simulink model "observer_based_SF_controller"  (R2017b)
settings: Solver=VariableStepAuto  StartTime=0.0  StopTime=10.0  RelTol=1e-3
values from neighbouring files (symbols this model uses):
  mA = [0 1 0; 0 -b/j k/j; 0 k/l -r/l]    [ProjectFile1.m]
  mB = [0;0; 1/l]    [ProjectFile1.m]
  mC = [1 0 0]    [ProjectFile1.m]
  mD = [0]    [ProjectFile1.m]
  mK = acker(mA, mB, desired_egnvalues)    [ProjectFile1.m]
  mL = acker(mA',mC', desired.ob.egnvalues)'    [ProjectFile1.m]
settings Model: Creator=insha  LastModifiedBy=insha

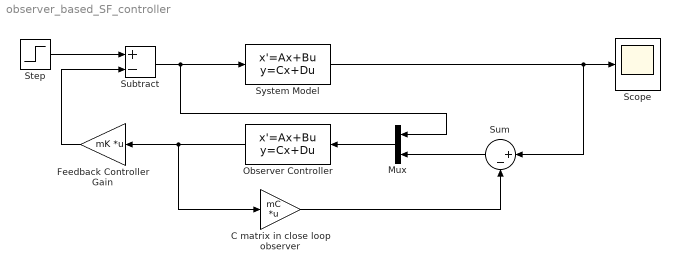
== system observer_based_SF_controller ==
  "C matrix in close loop observer " : Gain  Gain=mC  Multiplication=Matrix(K*u)
  Feedback Controller Gain : Gain  Gain=mK  Multiplication=Matrix(K*u)
  Mux : Mux  Inputs=2
  Observer Controller : StateSpace  A=mA  B=[mB mL]  C=[1 0 0; 0 1 0; 0 0 1]  D=[0 0; 0 0; 0 0]  InitialCondition=0
  Scope : Scope
  Step : Step  SampleTime=0
  Subtract : Sum  Inputs=+-
  Sum : Sum  Inputs=|+-
  "System Model " : StateSpace  A=mA  B=mB  C=mC  D=mD  InitialCondition=0
  wires:
  "System Model "/1 -> Sum/1, Scope/1
  Mux/1 -> Observer Controller/1
  Sum/1 -> Mux/2
  "C matrix in close loop observer "/1 -> Sum/2
  Observer Controller/1 -> "C matrix in close loop observer "/1, Feedback Controller Gain/1
  Feedback Controller Gain/1 -> Subtract/2
  Step/1 -> Subtract/1
  Subtract/1 -> Mux/1, "System Model "/1
